simulink model "exnb4137986_Q6"  (R2024b)
settings: Solver=FixedStepAuto  StartTime=0.0  StopTime=15  FixedStep=0.001  RelTol=1e-3
values from neighbouring files (symbols this model uses):
  A = double(subs(A, {x1, x2}, {m_star_2, omega_star_2}))    [exnb4137986_Q4_par.m]    (also in exnb4137986_Q6_par.m; exnb4137986_Q8_par.m; exnb4137986_Q9_par.m)
  B = diff(X_dot, u)    [exnb4137986_Q4_par.m]    (also in exnb4137986_Q6_par.m = double(diff(X_dot, u)); exnb4137986_Q8_par.m = double(diff(X_dot, u)); exnb4137986_Q9_par.m = double(diff(X_dot, u)))
  K = place(A, B, lambda_cl)    [exnb4137986_Q6_par.m]    (also in exnb4137986_Q8_par.m; exnb4137986_Q9_par.m)
  m_star_1 = double(subs(m, x2, omega_star_1))    [exnb4137986_Q4_par.m]    (also in exnb4137986_Q6_par.m; exnb4137986_Q8_par.m; exnb4137986_Q9_par.m)
  m_star_2 = double(subs(m, x2, omega_star_2))    [exnb4137986_Q4_par.m]    (also in exnb4137986_Q6_par.m; exnb4137986_Q8_par.m; exnb4137986_Q9_par.m)
  omega_star_1 = 200    [exnb4137986_Q4_par.m]    (also in exnb4137986_Q6_par.m; exnb4137986_Q8_par.m; exnb4137986_Q9_par.m)
  omega_star_2 = 300    [exnb4137986_Q4_par.m]    (also in exnb4137986_Q6_par.m; exnb4137986_Q8_par.m; exnb4137986_Q9_par.m)
  u_star_1 = double(subs(u, x2, omega_star_1))    [exnb4137986_Q4_par.m]    (also in exnb4137986_Q6_par.m; exnb4137986_Q8_par.m; exnb4137986_Q9_par.m)
  values = [1, 10, 0.1, 40]    [exnb4137986_Q4_par.m]    (also in exnb4137986_Q6_par.m; exnb4137986_Q8_par.m; exnb4137986_Q9_par.m)
settings Model: Creator=therkelsen  LastModifiedBy=therkelsen

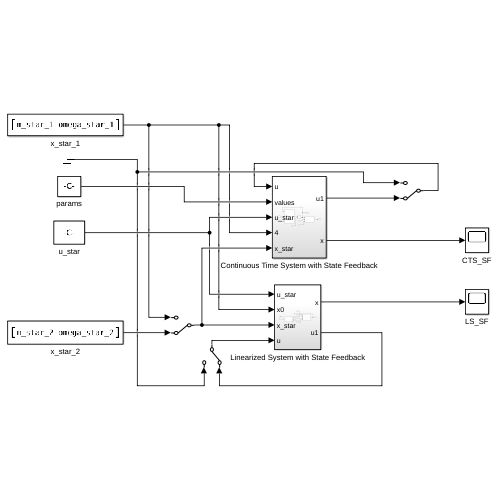
[thumbnail: Simulink's stored preview of the top-level diagram]
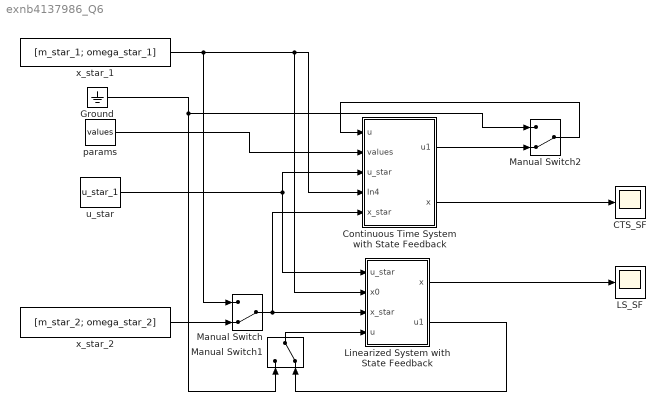
== system exnb4137986_Q6 ==
  CTS_SF : Scope
  Continuous Time System with State Feedback : Subsystem
  Ground : Ground
  LS_SF : Scope
  Linearized System with State Feedback : Subsystem
  Manual Switch : ManualSwitch  CurrentSetting=0
  Manual Switch1 : ManualSwitch  CurrentSetting=0
  Manual Switch2 : ManualSwitch  CurrentSetting=0
  params : Constant  Value=values
  u_star : Constant  Value=u_star_1
  x_star_1 : Constant  Value=[m_star_1; omega_star_1]
  x_star_2 : Constant  Value=[m_star_2; omega_star_2]
  wires:
  Linearized System with State Feedback/1(x) -> LS_SF/1
  Continuous Time System with State Feedback/1(u1) -> Manual Switch2/2
  Continuous Time System with State Feedback/2(x) -> CTS_SF/1
  Manual Switch1/1 -> Linearized System with State Feedback/4(u)
  Linearized System with State Feedback/2(u1) -> Manual Switch1/2
  Manual Switch/1 -> Linearized System with State Feedback/3(x_star), Continuous Time System with State Feedback/5(x_star)
  u_star/1 -> Linearized System with State Feedback/1(u_star), Continuous Time System with State Feedback/3(u_star)
  params/1 -> Continuous Time System with State Feedback/2(values)
  x_star_2/1 -> Manual Switch/2
  Ground/1 -> Manual Switch1/1, Manual Switch2/1
  Manual Switch2/1 -> Continuous Time System with State Feedback/1(u)
  x_star_1/1 -> Continuous Time System with State Feedback/4(In4), Linearized System with State Feedback/2(x0), Manual Switch/1

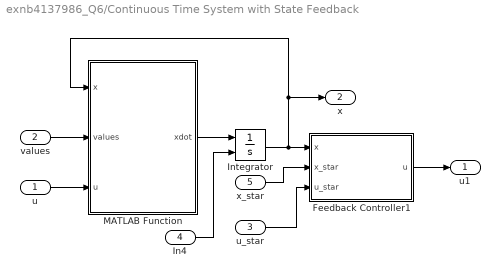
== system exnb4137986_Q6/Continuous Time System with State Feedback ==
  u : Inport
  values : Inport  Port=2
  u_star : Inport  Port=3
  In4 : Inport  Port=4
  x_star : Inport  Port=5
  Feedback Controller1 : Subsystem
  Integrator : Integrator  InitialConditionSource=external
  MATLAB Function : MATLAB Function  TreatAsAtomicUnit=on
  u1 : Outport
  x : Outport  Port=2
  wires:
  Feedback Controller1/1(u) -> u1/1
  Integrator/1 -> x/1, MATLAB Function/1(x), Feedback Controller1/1(x)
  In4/1 -> Integrator/2
  u_star/1 -> Feedback Controller1/3(u_star)
  x_star/1 -> Feedback Controller1/2(x_star)
  MATLAB Function/1(xdot) -> Integrator/1
  u/1 -> MATLAB Function/3(u)
  values/1 -> MATLAB Function/2(values)

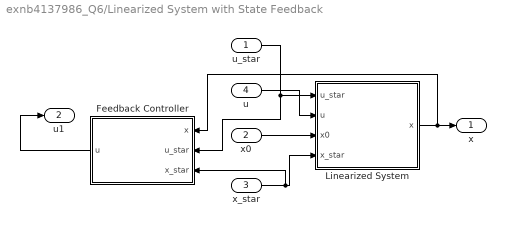
== system exnb4137986_Q6/Linearized System with State Feedback ==
  u_star : Inport
  x0 : Inport  Port=2
  x_star : Inport  Port=3
  u : Inport  Port=4
  Feedback Controller : Subsystem
  Linearized System : Subsystem
  x : Outport
  u1 : Outport  Port=2
  wires:
  Linearized System/1(x) -> x/1, Feedback Controller/1(x)
  x0/1 -> Linearized System/3(x0)
  u/1 -> Linearized System/2(u)
  x_star/1 -> Linearized System/4(x_star), Feedback Controller/3(x_star)
  u_star/1 -> Linearized System/1(u_star), Feedback Controller/2(u_star)
  Feedback Controller/1(u) -> u1/1

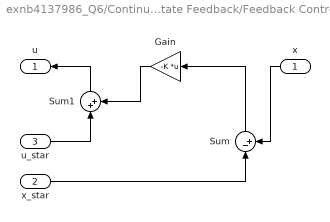
== system exnb4137986_Q6/Continuous Time System with State Feedback/Feedback Controller1 ==
  x : Inport
  x_star : Inport  Port=2
  u_star : Inport  Port=3
  Gain : Gain  Gain=-K  Multiplication=Matrix(K*u)
  Sum : Sum  Inputs=|-+
  Sum1 : Sum  Inputs=|++
  u : Outport
  wires:
  x/1 -> Sum/2
  Gain/1 -> Sum1/2
  Sum/1 -> Gain/1
  x_star/1 -> Sum/1
  u_star/1 -> Sum1/1
  Sum1/1 -> u/1

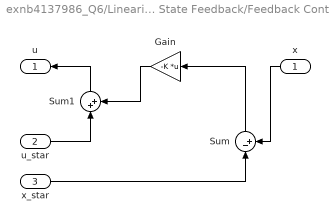
== system exnb4137986_Q6/Linearized System with State Feedback/Feedback Controller ==
  x : Inport
  u_star : Inport  Port=2
  x_star : Inport  Port=3
  Gain : Gain  Gain=-K  Multiplication=Matrix(K*u)
  Sum : Sum  Inputs=|-+
  Sum1 : Sum  Inputs=|++
  u : Outport
  wires:
  x/1 -> Sum/2
  Gain/1 -> Sum1/2
  Sum/1 -> Gain/1
  x_star/1 -> Sum/1
  u_star/1 -> Sum1/1
  Sum1/1 -> u/1

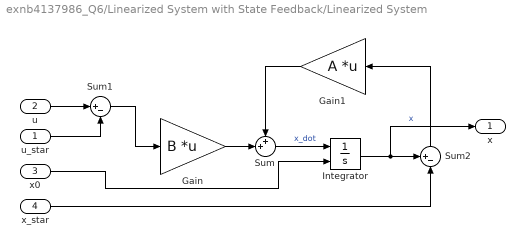
== system exnb4137986_Q6/Linearized System with State Feedback/Linearized System ==
  u_star : Inport
  u : Inport  Port=2
  x0 : Inport  Port=3
  x_star : Inport  Port=4
  Gain : Gain  Gain=B  Multiplication=Matrix(K*u) (u vector)
  Gain1 : Gain  Gain=A  Multiplication=Matrix(K*u) (u vector)
  Integrator : Integrator  InitialConditionSource=external  InitialCondition=[0.5;0]
  Sum : Sum  Inputs=++|
  Sum1 : Sum  Inputs=|+-
  Sum2 : Sum  Inputs=+-|
  x : Outport
  wires:
  Sum/1 -> Integrator/1  "x_dot"
  Gain1/1 -> Sum/1
  u/1 -> Sum1/1
  Gain/1 -> Sum/2
  Integrator/1 -> x/1, Sum2/1  "x"
  x_star/1 -> Sum2/2
  u_star/1 -> Sum1/2
  Sum1/1 -> Gain/1
  Sum2/1 -> Gain1/1
  x0/1 -> Integrator/2

== matlab function exnb4137986_Q6/Continuous Time System with State Feedback/MATLAB Function ==
  data: x input; values input; u input; xdot output
function xdot = fcn(x, values, u)

q1 = values(1);
q2 = values(2);
q3 = values(3);
J = values(4);

xdot = [-q1*x(2)*x(1) + u;
         q2/J*x(1) - q3/J*x(2)];
